simulink model "Simulank"  (R2022b)
settings: Solver=VariableStepAuto  StartTime=0.0  StopTime=30  MaxStep=0.001  RelTol=1e-3
settings Model: Creator=ahmed  LastModifiedBy=ahmed

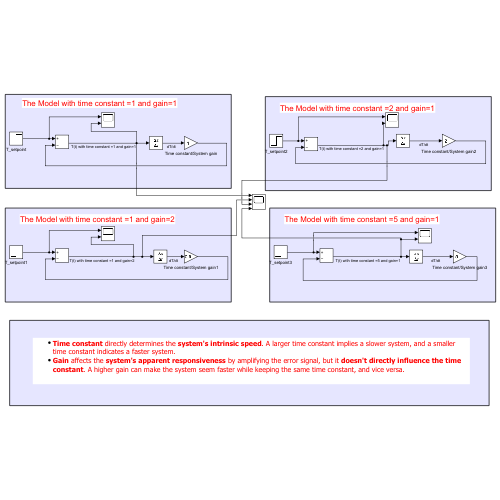
[thumbnail: Simulink's stored preview of the top-level diagram]
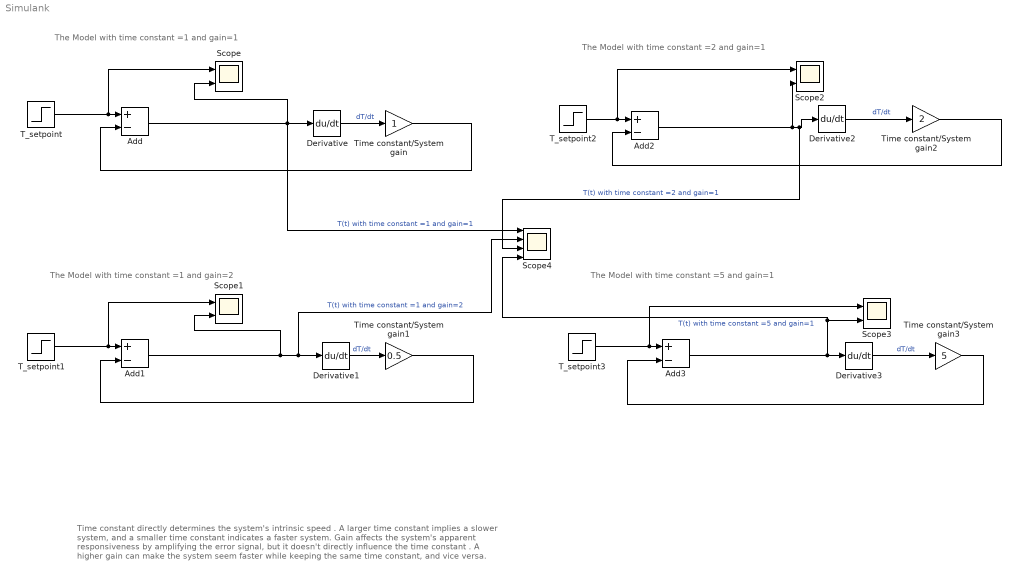
== system Simulank ==
  note: The Model with time constant =1 and gain=1
  note: The Model with time constant =1 and gain=2
  note: The Model with time constant =2 and gain=1
  note: The Model with time constant =5 and gain=1
  note: Time constant directly determines the system's intrinsic speed . A larger time constant implies a slower system, and a smaller time constant indicates a faster system.
      | Gain affects the system's apparent responsiveness by amplifying the error signal, but it doesn't directly influence the time constant . A higher gain can make the system seem faster while keeping the same time constant, and vice versa.
  Add{,1..3} (4 alike) : Sum  Inputs=+-
  Derivative{,1..3} (4 alike) : Derivative
  Scope{,1..3} (4 alike) : Scope  NumInputPorts=2
  Scope4 : Scope  NumInputPorts=4
  T_setpoint{,1..3} (4 alike) : Step  Time=2  SampleTime=0
  Time constant/System gain : Gain
  Time constant/System gain1 : Gain  Gain=0.5
  Time constant/System gain2 : Gain  Gain=2
  Time constant/System gain3 : Gain  Gain=5
  wires:
  Add/1 -> Scope/2, Scope4/1, Derivative/1  "T(t) with time constant =1 and gain=1"
  Derivative/1 -> Time constant/System gain/1  "dT/dt"
  Time constant/System gain/1 -> Add/2
  T_setpoint/1 -> Scope/1, Add/1
  Derivative1/1 -> Time constant/System gain1/1  "dT/dt"
  T_setpoint1/1 -> Scope1/1, Add1/1
  Time constant/System gain1/1 -> Add1/2
  Add1/1 -> Scope1/2, Scope4/2, Derivative1/1  "T(t) with time constant =1 and gain=2"
  Derivative2/1 -> Time constant/System gain2/1  "dT/dt"
  T_setpoint2/1 -> Scope2/1, Add2/1
  Time constant/System gain2/1 -> Add2/2
  Add2/1 -> Scope4/3, Derivative2/1, Scope2/2  "T(t) with time constant =2 and gain=1"
  Derivative3/1 -> Time constant/System gain3/1  "dT/dt"
  T_setpoint3/1 -> Scope3/1, Add3/1
  Time constant/System gain3/1 -> Add3/2
  Add3/1 -> Scope3/2, Scope4/4, Derivative3/1  "T(t) with time constant =5 and gain=1"
